simulink model "TP09_Ej07"  (R2020b)
settings: Solver=FixedStepAuto  StartTime=0.0  StopTime=2.5  FixedStep=1e-3  RelTol=1e-3
settings Model: Creator=Juan  LastModifiedBy=Juan

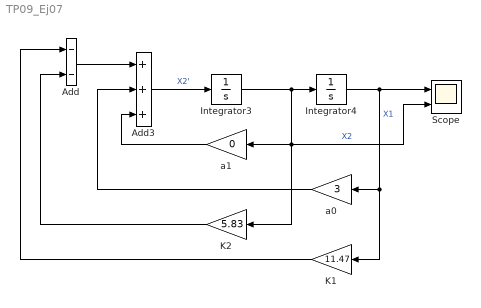
== system TP09_Ej07 ==
  Add : Sum  Inputs=--
  Add3 : Sum  Inputs=+++
  Integrator3 : Integrator  InitialCondition=1
  Integrator4 : Integrator  InitialCondition=-1
  K1 : Gain  Gain=11.47
  K2 : Gain  Gain=5.83
  Scope : Scope  NumInputPorts=2
  a0 : Gain  Gain=3
  a1 : Gain  Gain=0
  wires:
  Integrator4/1 -> K1/1, a0/1, Scope/1  "X1"
  Integrator3/1 -> K2/1, Scope/2, a1/1, Integrator4/1  "X2"
  Add3/1 -> Integrator3/1  "X2'"
  a1/1 -> Add3/3
  a0/1 -> Add3/2
  K1/1 -> Add/1
  K2/1 -> Add/2
  Add/1 -> Add3/1
